simulink subsystem "State_Machine"  (R2024b)
settings: Solver=VariableStepAuto  StartTime=0.0  StopTime=10.0  RelTol=1e-3
values from neighbouring files (symbols this model uses):
  vehicle = Vehicle(100000,30,60,deg2rad(20),800000,2000000, Name = "Default")    [CasADi_MPC.m]
settings Model: Creator=alexa  LastModifiedBy=thatf

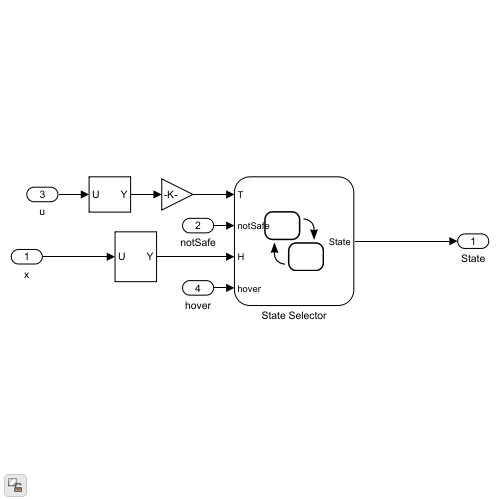
[thumbnail: Simulink's stored preview of the top-level diagram]
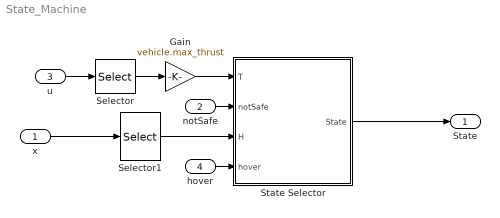
== system State_Machine ==
  x : Inport
  notSafe : Inport  Port=2
  u : Inport  Port=3
  hover : Inport  Port=4
  Gain : Gain  Gain=vehicle.max_thrust
  Selector : Selector  InputPortWidth=dof.nu  IndexOptions=Index vector (dialog)  Indices=[1]  OutputSizes=1
  Selector1 : Selector  InputPortWidth=dof.nx  IndexOptions=Index vector (dialog)  Indices=[2]  OutputSizes=1
  State Selector : Stateflow chart  TreatAsAtomicUnit=on
  State : Outport
  wires:
  State Selector/1(State) -> State/1
  notSafe/1 -> State Selector/2(notSafe)
  hover/1 -> State Selector/4(hover)
  u/1 -> Selector/1
  Selector/1 -> Gain/1
  Gain/1 -> State Selector/1(T)
  x/1 -> Selector1/1
  Selector1/1 -> State Selector/3(H)

== stateflow chart State_Machine/State Selector ==
  state Landed
  state FollowPlan
  state EmergencyLanding
  state Hover
  (default) -> Landed
  Landed -> FollowPlan : [T > W || H > 0]
  Hover -> FollowPlan [order 1] : [hover == 0]
  FollowPlan -> Hover [order 2] : [hover == 1]
  FollowPlan -> EmergencyLanding [order 1] : [notSafe == 1]
  Hover -> EmergencyLanding [order 2] : [notSafe == 1]
  data: T input; W constant double =vehicle.m * g; notSafe input; State output Enum: StateEnum; H input; hover input
